simulink model "verify_Pressure_Drop_PipeTheory_mdl"  (R2016b)
settings: Solver=VariableStepDiscrete  StartTime=0.0  StopTime=10  MaxStep=1  RelTol=1e-3  EnableMultiTasking=on
libraries: carnot x2
settings Model: Creator=drhf  LastModifiedBy=drhf
settings DataIOCC: LimitDataPoints=on  SaveFormat=Array  SignalLoggingSaveFormat=ModelDataLogs
settings OptimizationCC: ExpressionDepthLimit=2147483647  LifeSpan=inf
settings DebuggingCC: UnderspecifiedInitializationDetection=Classic  MergeDetectMultiDrivingBlocksExec=none  SolverPrmCheckMsg=warning  FcnCallInpInsideContextMsg=warning  StateNameClashWarn=warning  SFUnexpectedBacktrackingDiag=warning  SFNoUnconditionalDefaultTransitionDiag=warning  SFExecutionAtInitializationDiag=none
settings HardwareCC: ProdBitPerPointer=32  ProdBitPerSizeT=32  ProdBitPerPtrDiffT=32  ProdLargestAtomicFloat=None  ProdIntDivRoundTo=Undefined  ProdEndianess=Unspecified  ProdWordSize=32  ProdHWDeviceType=32-bit Generic
settings ModelReferenceCC: PropagateSignalLabelsOutOfModel=off
settings GRTTargetCC: TargetLangStandard=C89/C90 (ANSI)  GeneratePreprocessorConditionals=Disable all  CombineOutputUpdateFcns=off  GRTInterface=on
settings ConfigComp: CovMetricSettings=dw  CovHtmlReporting=on  CovSaveCumulativeToWorkspaceVar=on  CovSaveSingleToWorkspaceVar=on  CovExternalEMLEnable=off

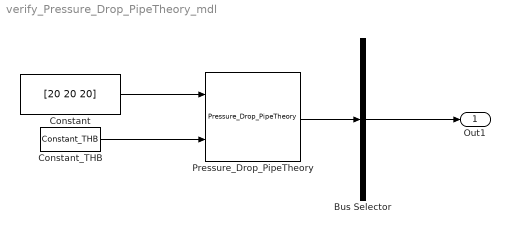
== system verify_Pressure_Drop_PipeTheory_mdl ==
  Bus Selector : BusSelector  OutputSignals=Pressure,GeodeticHeight  OutputAsBus=on
  Constant : Constant  Value=[20 20 20]
  Constant_THB : carnot/Source/Simple/Constant_THB  t=40  mdot=200/3600  p=2e5  mID=Full Pressure Drop with Static Height  fluid=Water  mix=0  mix2=0  mix3=0  dia=0.02  hgt=0
  Pressure_Drop_PipeTheory : carnot/Basic/Pressure_Drop/Pressure_Drop_PipeTheory  dia=0.02  len=1  rough=0.04  nbend=1
  Out1 : Outport
  wires:
  Constant_THB/1 -> Pressure_Drop_PipeTheory/2
  Pressure_Drop_PipeTheory/1 -> Bus Selector/1
  Bus Selector/1 -> Out1/1
  Constant/1 -> Pressure_Drop_PipeTheory/1
